simulink model "case_9_ego_stopped_lead_accelerating"  (R2025b)
settings: Solver=VariableStepAuto  StartTime=0.0  StopTime=10.0  RelTol=1e-3
settings Model: Creator=sanborkl  LastModifiedBy=admin

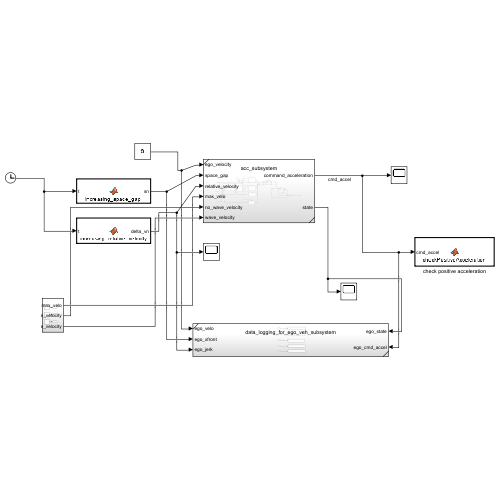
[thumbnail: Simulink's stored preview of the top-level diagram]
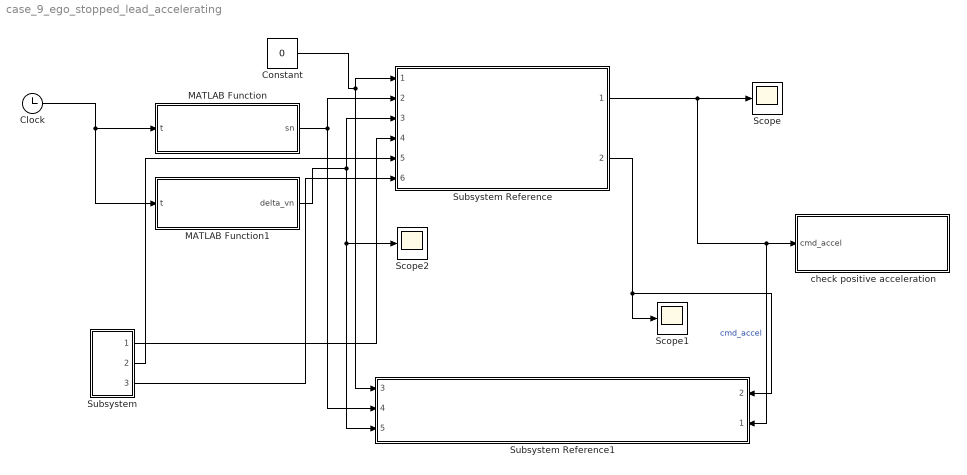
== system case_9_ego_stopped_lead_accelerating ==
  Clock : Clock
  Constant : Constant  Value=0
  MATLAB Function : MATLAB Function  TreatAsAtomicUnit=on
  MATLAB Function1 : MATLAB Function  TreatAsAtomicUnit=on
  Scope : Scope
      settings: ActiveDisplayYMinimum=0.49999999999999994  ActiveDisplayYMaximum=2.5
  Scope1 : Scope
      settings: ActiveDisplayYMinimum=-0.0532339983076785  ActiveDisplayYMaximum=1.2927998690958942
  Scope2 : Scope
      settings: ActiveDisplayYMinimum=-2.4999999999999996  ActiveDisplayYMaximum=22.5  DataLoggingVariableName=ScopeData2
  Subsystem : Subsystem
  Subsystem Reference : Subsystem  ReferencedSubsystem=acc_subsystem
  Subsystem Reference1 : Subsystem  ReferencedSubsystem=data_logging_for_ego_veh_subsystem
      settings: PortSchema="{\"entries\":[{\"content\":{\"sides\":[{\"content\":{\"connectorIds\":[\"In3\",\"In4\",\"In5\"]},\"type\":\"ConnectorPlacement.EquallySpacedRectSide\",\"uuid\":\"0b96bcaa-a470-46c9-9268-f4bd6b1035a8\"},{\"content\":{\"connectorIds\":[\"In2\",\"In1\"],\"side\":\"RIGHT\"},\"type\":\"ConnectorPlacement.EquallySpacedRectSide\",\"uuid\":\"8e49005a-1e53-4e76-b163-50df0eb9f2cc\"},{\"content\":{\"side\":\"TOP\"},\"type\":\"ConnectorPlacement.EquallySpacedRectSide\",\"uuid\":\"3ff4af65-efca-4a64-9b7f-f479498e89e2\"}]},\"type\":\"ConnectorPlacement.EquallySpacedConnector\",\"uuid\":\"f10caef7-9599-4d5c-a8fd-3eb49f6fcaa8\"}],\"packageUris\":[\"http://schema.mathworks.com/mf0/Connector/R2020b\"],\"version\":\"1.0\"}"
  check positive acceleration : MATLAB Function  TreatAsAtomicUnit=on
  wires:
  MATLAB Function1/1(delta_vn) -> Subsystem Reference1/5, Scope2/1, Subsystem Reference/3
  MATLAB Function/1(sn) -> Subsystem Reference1/4, Subsystem Reference/2
  Constant/1 -> Subsystem Reference1/3, Subsystem Reference/1
  Clock/1 -> MATLAB Function1/1(t), MATLAB Function/1(t)
  Subsystem Reference/2 -> Subsystem Reference1/2, Scope1/1
  Subsystem Reference/1 -> Subsystem Reference1/1, check positive acceleration/1(cmd_accel), Scope/1  "cmd_accel"
  Subsystem/1(max_velo) -> Subsystem Reference/4
  Subsystem/2(no_wave_velocity) -> Subsystem Reference/5
  Subsystem/3(wave_velocity) -> Subsystem Reference/6

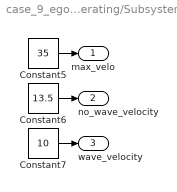
== system case_9_ego_stopped_lead_accelerating/Subsystem ==
  Constant5 : Constant  Value=35
  Constant6 : Constant  Value=13.5
  Constant7 : Constant  Value=10
  max_velo : Outport
  no_wave_velocity : Outport  Port=2
  wave_velocity : Outport  Port=3
  wires:
  Constant7/1 -> wave_velocity/1
  Constant6/1 -> no_wave_velocity/1
  Constant5/1 -> max_velo/1

== matlab function case_9_ego_stopped_lead_accelerating/MATLAB Function1 ==
  data: t input; delta_vn output
function delta_vn = increasing_relative_velocity(t)

delta_vn = 2 * t;

== matlab function case_9_ego_stopped_lead_accelerating/check positive acceleration ==
  data: cmd_accel input
function checkPositiveAcceleration(cmd_accel)
%#codegen
coder.extrinsic('disp', 'sprintf');

if cmd_accel < 0
    msg = sprintf('Error: Negative command acceleration: %.3f, should be positive', ...
                  cmd_accel);
    disp(msg);
end
end

== matlab function case_9_ego_stopped_lead_accelerating/MATLAB Function ==
  data: t input; sn output
function sn = increasing_space_gap(t)

sn = 3 * t + 20;
